simulink model "ARI_26_7_stability_1st_order"  (Simulink 7.8)
settings: Solver=ode45  StartTime=0.0  StopTime=0.5  RelTol=1e-3
libraries: simulink x1
settings Model: Creator=Michael Sebek  ModifiedByFormat=Michael Sebek  LastModifiedBy=Michael Sebek
settings OptimizationCC: InitFltsAndDblsToZero=on
settings DebuggingCC: SaveWithParameterizedLinksMsg=none  SignalResolutionControl=TryResolveAllWithWarning  MultiTaskDSMMsg=warning  MultiTaskCondExecSysMsg=none  FcnCallInpInsideContextMsg=Use local settings  StrictBusMsg=None
settings RTWCC: IncludeERTFirstTime=on
settings GRTTargetCC: TargetFcnLib=ansi_tfl_tmw.mat

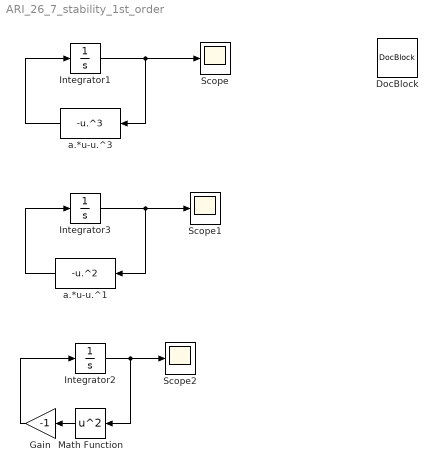
== system ARI_26_7_stability_1st_order ==
  DocBlock : simulink/Model-Wide Utilities/DocBlock  DocumentType=Text
      content=|
      | %  délka simulace = .5
      | %  ignorovat hlášení
  Gain : Gain  Gain=-1
  Integrator1 : Integrator  InitialCondition=[-2,-1.5,-1,-0.5,-0.1,0,0.1,0.5,1,1.5,2]
  Integrator2 : Integrator  InitialCondition=[-2,-1.5,-1,-0.5,-0.1,0,0.1,0.5,1,1.5,2]
  Integrator3 : Integrator  InitialCondition=[-2,-1.5,-1,-0.5,-0.1,0,0.1,0.5,1,1.5,2]
  Math Function : Math  Operator=square  SaturateOnIntegerOverflow=on
  Scope : Scope
      settings: TimeRange=0.5  YMin=-3  YMax=3
  Scope1 : Scope
      settings: TimeRange=0.5  YMax=3
  Scope2 : Scope
      settings: TimeRange=0.5  YMax=3  SaveName=ScopeData2
  a.*u-u.^1 : MATLABFcn  MATLABFcn=-u.^2
      mask Display: disp('-u.^2')
  a.*u-u.^3 : MATLABFcn  MATLABFcn=-u.^3
      mask Display: disp('-u.^3')
  wires:
  Integrator2/1 -> Math Function/1, Scope2/1
  Math Function/1 -> Gain/1
  Gain/1 -> Integrator2/1
  a.*u-u.^3/1 -> Integrator1/1
  Integrator1/1 -> Scope/1, a.*u-u.^3/1
  a.*u-u.^1/1 -> Integrator3/1
  Integrator3/1 -> Scope1/1, a.*u-u.^1/1
